simulink subsystem "joystick_to_pwm"  (R2025b)
settings: Solver=VariableStepAuto  StartTime=0.0  StopTime=10.0  RelTol=1e-3
settings Model: Creator=vulcangrip  LastModifiedBy=vulcangrip

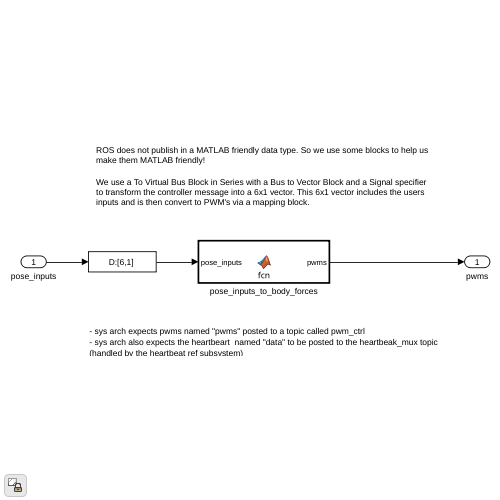
[thumbnail: Simulink's stored preview of the top-level diagram]
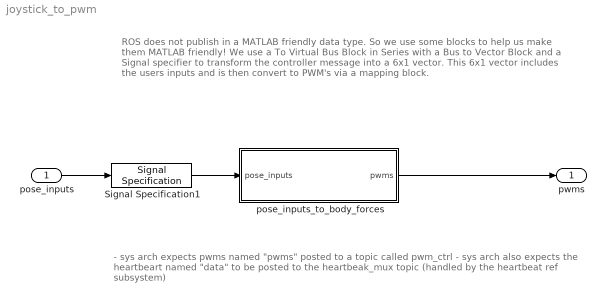
== system joystick_to_pwm ==
  note: - sys arch expects pwms named "pwms" posted to a topic called pwm_ctrl
      | - sys arch also expects the heartbeart  named "data" to be posted to the heartbeak_mux topic (handled by the heartbeat ref subsystem)
  note: ROS does not publish in a MATLAB friendly data type. So we use some blocks to help us make them MATLAB friendly!
      |
      | We use a To Virtual Bus Block in Series with a Bus to Vector Block and a Signal specifier to transform the controller message into a 6x1 vector. This 6x1 vector includes the users inputs and is then convert to PWM's via a mapping block.
  pose_inputs : Inport
  Signal Specification1 : SignalSpecification  Dimensions=[6,1]
  pose_inputs_to_body_forces : MATLAB Function  TreatAsAtomicUnit=on
  pwms : Outport
  wires:
  Signal Specification1/1 -> pose_inputs_to_body_forces/1(pose_inputs)
  pose_inputs/1 -> Signal Specification1/1
  pose_inputs_to_body_forces/1(pwms) -> pwms/1

== matlab function joystick_to_pwm/pose_inputs_to_body_forces ==
  data: pwms output; pose_inputs input
function pwms = fcn(pose_inputs)

[pwms_vert,pwms_horiz] = pose_inputs_to_body_forces(pose_inputs);

pwms = int32([pwms_vert,pwms_horiz])';
